simulink model "guidance_fuzzy_alt"  (R2017b)
settings: Solver=FixedStepDiscrete  StartTime=0.0  StopTime=inf  FixedStep=0.01  RelTol=1e-3
model workspace (MAT data in the model file):
  SL_ROS_VariableLengthArrays_MaxSizes : struct (value not decoded)
undefined symbols (not defined in the file): Data, Data_SL_Info
libraries: dspstat3 x14, robotlib x10, simulink_extras x7, simulink x4, dspswit3 x1
(part 2 of 2)

== system guidance_fuzzy_alt/pixel_per_sec_to_m_per_sec ==
  height : Inport
  vx(pix/sec) : Inport  Port=2
  vy(pix/sec) : Inport  Port=3
  Product : Product
  Product1 : Product
  camera_trigonometric_factor(m/pix) : Constant  Value=342.85
  of_vx_Divide : Product  Inputs=*/
  of_vy_Divide : Product  Inputs=*/
  vx_Moving Average : dspstat3/Moving Average  Method=Sliding window  SpecifyWindowLength=on  WindowLength=35  ForgettingFactor=0.9  SimulateUsing=Code generation
  vy_Moving Average : dspstat3/Moving Average  Method=Sliding window  SpecifyWindowLength=on  WindowLength=35  ForgettingFactor=0.9  SimulateUsing=Code generation
  vx(m/s) : Outport
  vy(m/s) : Outport  Port=2
  wires:
  height/1 -> Product1/1, Product/1
  of_vx_Divide/1 -> vx_Moving Average/1
  Product/1 -> of_vy_Divide/1
  Product1/1 -> of_vx_Divide/1
  vy_Moving Average/1 -> vy(m/s)/1
  vx_Moving Average/1 -> vx(m/s)/1
  of_vy_Divide/1 -> vy_Moving Average/1
  vy(pix/sec)/1 -> Product1/2
  camera_trigonometric_factor(m/pix)/1 -> of_vy_Divide/2, of_vx_Divide/2
  vx(pix/sec)/1 -> Product/2

== system guidance_fuzzy_alt/throttle_handler_climb_mode ==
  desired_throttle : Inport
  height : Inport  Port=2
  landing : Inport  Port=3
  If Action Subsystem4 : Subsystem  TreatAsAtomicUnit=on
  If Action Subsystem5 : Subsystem  TreatAsAtomicUnit=on
  If2 : If  IfExpression=u1 == 1  ElseIfExpressions=u1 == 0  ShowElse=off
  Merge2 : Merge
  Z_command : Scope
  throttle : Outport
  wires:
  height/1 -> If Action Subsystem4/1(In2)
  If Action Subsystem5/1(Out1) -> Merge2/2
  If Action Subsystem4/1(Out1) -> Merge2/1
  landing/1 -> If2/1
  Merge2/1 -> Z_command/1, throttle/1
  If2/1 -> If Action Subsystem4/Action
  If2/2 -> If Action Subsystem5/Action
  desired_throttle/1 -> If Action Subsystem5/1(In1)

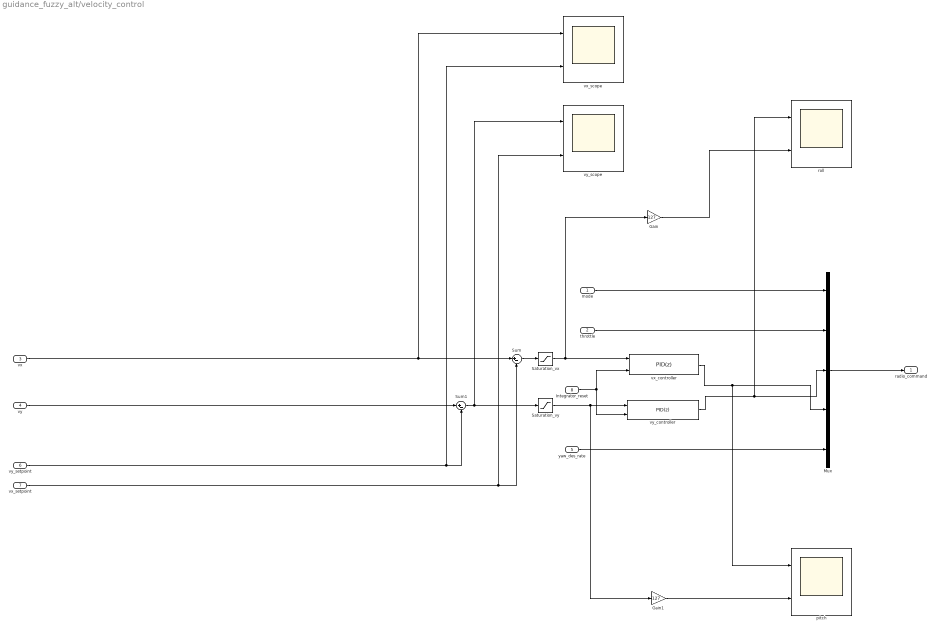
== system guidance_fuzzy_alt/velocity_control ==
  mode : Inport
  throttle : Inport  Port=2
  vx : Inport  Port=3
  vy : Inport  Port=4
  yaw_des_rate : Inport  Port=5
  vy_setpoint : Inport  Port=6
  vx_setpoint : Inport  Port=7
  Integrator_reset : Inport  Port=8
  Gain : Gain  Gain=127
  Gain1 : Gain  Gain=127
  Mux : Mux  Inputs=5
  Saturation_vx : Saturate  UpperLimit=1  LowerLimit=-1
  Saturation_vy : Saturate  UpperLimit=1  LowerLimit=-1
  Sum : Sum  Inputs=|+-
  Sum1 : Sum  Inputs=|+-
  pitch : Scope  NumInputPorts=2
  roll : Scope  NumInputPorts=2
  vx_controller : simulink/Continuous/PID Controller  Controller=PID  TimeDomain=Discrete-time  SampleTime=-1  IntegratorMethod=Forward Euler  FilterMethod=Forward Euler  Form=Parallel  UseFilter=on  ControllerParametersSource=internal  P=40  I=30  D=1  N=100  InitialConditionSource=internal  InitialConditionForIntegrator=0  InitialConditionForFilter=0  ExternalReset=either  LimitOutput=on  UpperSaturationLimit=127  LowerSaturationLimit=-127  LinearizeAsGain=off  AntiWindupMode=none  Kb=1  TrackingMode=off  Kt=1  PParamMin=[]  PParamMax=[]  IParamMin=[]  IParamMax=[]  DParamMin=[]  DParamMax=[]  NParamMin=[]  NParamMax=[]  KbParamMin=[]  KbParamMax=[]  KtParamMin=[]  KtParamMax=[]  POutMin=[]  POutMax=[]  IOutMin=[]  IOutMax=[]  DOutMin=[]  DOutMax=[]  NOutMin=[]  NOutMax=[]  KbOutMin=[]  KbOutMax=[]  KtOutMin=[]  KtOutMax=[]  IntegratorOutMin=[]  IntegratorOutMax=[]  FilterOutMin=[]  FilterOutMax=[]  SumOutMin=[]  SumOutMax=[]  SumI1OutMin=[]  SumI1OutMax=[]  SumI2OutMin=[]  SumI2OutMax=[]  SumI3OutMin=[]  SumI3OutMax=[]  SumDOutMin=[]  SumDOutMax=[]  SaturationOutMin=[]  SaturationOutMax=[]  IntegratorContinuousStateAttributes=''  IntegratorStateMustResolveToSignalObject=off  IntegratorRTWStateStorageClass=Auto  FilterContinuousStateAttributes=''  FilterStateMustResolveToSignalObject=off  FilterRTWStateStorageClass=Auto  DifferentiatorICPrevScaledInput=0  DifferentiatorOutMin=[]  DifferentiatorOutMax=[]  InitialConditionSetting=State (most efficient)  FilterDiffOutCoefMin=[]  FilterDiffOutCoefMax=[]  SumDenOutMin=[]  SumDenOutMax=[]  SumNumOutMin=[]  SumNumOutMax=[]  ReciprocalOutMin=[]  ReciprocalOutMax=[]  DivideOutMin=[]  DivideOutMax=[]  TunerSelectOption=Transfer Function Based (PID Tuner App)
  vx_scope : Scope  NumInputPorts=2
  vy_controller : simulink/Continuous/PID Controller  Controller=PID  TimeDomain=Discrete-time  SampleTime=-1  IntegratorMethod=Forward Euler  FilterMethod=Forward Euler  Form=Parallel  UseFilter=on  ControllerParametersSource=internal  P=40  I=30  D=1  N=100  InitialConditionSource=internal  InitialConditionForIntegrator=0  InitialConditionForFilter=0  ExternalReset=either  LimitOutput=on  UpperSaturationLimit=127  LowerSaturationLimit=-127  LinearizeAsGain=off  AntiWindupMode=none  Kb=1  TrackingMode=off  Kt=1  PParamMin=[]  PParamMax=[]  IParamMin=[]  IParamMax=[]  DParamMin=[]  DParamMax=[]  NParamMin=[]  NParamMax=[]  KbParamMin=[]  KbParamMax=[]  KtParamMin=[]  KtParamMax=[]  POutMin=[]  POutMax=[]  IOutMin=[]  IOutMax=[]  DOutMin=[]  DOutMax=[]  NOutMin=[]  NOutMax=[]  KbOutMin=[]  KbOutMax=[]  KtOutMin=[]  KtOutMax=[]  IntegratorOutMin=[]  IntegratorOutMax=[]  FilterOutMin=[]  FilterOutMax=[]  SumOutMin=[]  SumOutMax=[]  SumI1OutMin=[]  SumI1OutMax=[]  SumI2OutMin=[]  SumI2OutMax=[]  SumI3OutMin=[]  SumI3OutMax=[]  SumDOutMin=[]  SumDOutMax=[]  SaturationOutMin=[]  SaturationOutMax=[]  IntegratorContinuousStateAttributes=''  IntegratorStateMustResolveToSignalObject=off  IntegratorRTWStateStorageClass=Auto  FilterContinuousStateAttributes=''  FilterStateMustResolveToSignalObject=off  FilterRTWStateStorageClass=Auto  DifferentiatorICPrevScaledInput=0  DifferentiatorOutMin=[]  DifferentiatorOutMax=[]  InitialConditionSetting=State (most efficient)  FilterDiffOutCoefMin=[]  FilterDiffOutCoefMax=[]  SumDenOutMin=[]  SumDenOutMax=[]  SumNumOutMin=[]  SumNumOutMax=[]  ReciprocalOutMin=[]  ReciprocalOutMax=[]  DivideOutMin=[]  DivideOutMax=[]  TunerSelectOption=Transfer Function Based (PID Tuner App)
  vy_scope : Scope  NumInputPorts=2
  radio_command : Outport
  wires:
  vy/1 -> Sum1/1
  vy_setpoint/1 -> vx_scope/2, Sum1/2
  Sum1/1 -> Saturation_vy/1, vy_scope/1
  vy_controller/1 -> roll/1, Mux/3
  Mux/1 -> radio_command/1
  vx/1 -> vx_scope/1, Sum/1
  Sum/1 -> Saturation_vx/1
  vx_setpoint/1 -> vy_scope/2, Sum/2
  mode/1 -> Mux/1
  yaw_des_rate/1 -> Mux/5
  throttle/1 -> Mux/2
  vx_controller/1 -> pitch/1, Mux/4
  Integrator_reset/1 -> vy_controller/2, vx_controller/2
  Saturation_vx/1 -> Gain/1, vx_controller/1
  Saturation_vy/1 -> Gain1/1, vy_controller/1
  Gain/1 -> roll/2
  Gain1/1 -> pitch/2

== system guidance_fuzzy_alt/DataChangeTimer/If Action Subsystem ==
  In1 : Inport
  Action Port : ActionPort  ActionType=then
  Out1 : Outport
  wires:
  In1/1 -> Out1/1

== system guidance_fuzzy_alt/DataChangeTimer/If Action Subsystem1 ==
  In1 : Inport
  Action Port : ActionPort  ActionType=else
  Out1 : Outport
  wires:
  In1/1 -> Out1/1

== system guidance_fuzzy_alt/Subsystem/If Action Subsystem16 ==
  In1 : Inport
  Action Port : ActionPort  ActionType=else
  Out1 : Outport
  wires:
  In1/1 -> Out1/1

== system guidance_fuzzy_alt/Subsystem/If Action Subsystem9 ==
  In1 : Inport
  Action Port : ActionPort  ActionType=then
  Out1 : Outport
  wires:
  In1/1 -> Out1/1

== system guidance_fuzzy_alt/Subsystem/Switch Case Action Subsystem ==
  In1 : Inport
  Action Port : ActionPort  ActionType=case
  Out1 : Outport
  wires:
  In1/1 -> Out1/1

== system guidance_fuzzy_alt/Subsystem/Switch Case Action Subsystem1 ==
  In1 : Inport
  Action Port : ActionPort  ActionType=case
  Out1 : Outport
  wires:
  In1/1 -> Out1/1

== system guidance_fuzzy_alt/Subsystem/Switch Case Action Subsystem2 ==
  In1 : Inport
  Action Port : ActionPort  ActionType=case
  Out1 : Outport
  wires:
  In1/1 -> Out1/1

== system guidance_fuzzy_alt/Subsystem/Switch Case Action Subsystem3 ==
  In1 : Inport
  Action Port : ActionPort  ActionType=case
  Out1 : Outport
  wires:
  In1/1 -> Out1/1

== system guidance_fuzzy_alt/Subsystem2/If Action Subsystem ==
  In1 : Inport
  Action Port : ActionPort  ActionType=then
  Out1 : Outport
  wires:
  In1/1 -> Out1/1

== system guidance_fuzzy_alt/Subsystem2/If Action Subsystem1 ==
  In1 : Inport
  Action Port : ActionPort  ActionType=elseif
  Out1 : Outport
  wires:
  In1/1 -> Out1/1

== system guidance_fuzzy_alt/Subsystem2/If Action Subsystem2 ==
  In1 : Inport
  Action Port : ActionPort  ActionType=else
  Out1 : Outport
  wires:
  In1/1 -> Out1/1

== system guidance_fuzzy_alt/Subsystem5/If Action Subsystem2 ==
  In1 : Inport
  Action Port : ActionPort  ActionType=then
  Out1 : Outport
  wires:
  In1/1 -> Out1/1

== system guidance_fuzzy_alt/Subsystem5/If Action Subsystem3 ==
  In1 : Inport
  Action Port : ActionPort  ActionType=else
  Out1 : Outport
  wires:
  In1/1 -> Out1/1

== system guidance_fuzzy_alt/Subsystem6/If Action Subsystem1 ==
  In1 : Inport
  Action Port : ActionPort  ActionType=then
  Out1 : Outport
  wires:
  In1/1 -> Out1/1

== system guidance_fuzzy_alt/Subsystem6/If Action Subsystem10 ==
  In1 : Inport
  Action Port : ActionPort  ActionType=then
  Selector : Selector  InputPortWidth=128  IndexOptions=Index vector (dialog)  Indices=[1:8]  OutputSizes=1
  Out1 : Outport
  wires:
  In1/1 -> Selector/1
  Selector/1 -> Out1/1

== system guidance_fuzzy_alt/Subsystem6/If Action Subsystem11 ==
  In1 : Inport
  Action Port : ActionPort  ActionType=then
  Selector : Selector  InputPortWidth=128  IndexOptions=Index vector (dialog)  Indices=[1:16]  OutputSizes=1
  Out1 : Outport
  wires:
  In1/1 -> Selector/1
  Selector/1 -> Out1/1

== system guidance_fuzzy_alt/Subsystem6/If Action Subsystem12 ==
  In1 : Inport
  Action Port : ActionPort  ActionType=then
  Selector : Selector  InputPortWidth=128  IndexOptions=Index vector (dialog)  Indices=[1:24]  OutputSizes=1
  Out1 : Outport
  wires:
  In1/1 -> Selector/1
  Selector/1 -> Out1/1

== system guidance_fuzzy_alt/Subsystem6/If Action Subsystem13 ==
  In1 : Inport
  Action Port : ActionPort  ActionType=then
  Out1 : Outport
  wires:
  In1/1 -> Out1/1

== system guidance_fuzzy_alt/Subsystem6/If Action Subsystem14 ==
  In1 : Inport
  Action Port : ActionPort  ActionType=then
  Out1 : Outport
  wires:
  In1/1 -> Out1/1

== system guidance_fuzzy_alt/Subsystem6/If Action Subsystem15 ==
  In1 : Inport
  Action Port : ActionPort  ActionType=then
  Out1 : Outport
  wires:
  In1/1 -> Out1/1

== system guidance_fuzzy_alt/Subsystem6/If Action Subsystem4 ==
  In1 : Inport
  Action Port : ActionPort  ActionType=then
  Out1 : Outport
  wires:
  In1/1 -> Out1/1

== system guidance_fuzzy_alt/Subsystem6/If Action Subsystem5 ==
  In1 : Inport
  Action Port : ActionPort  ActionType=then
  Out1 : Outport
  wires:
  In1/1 -> Out1/1

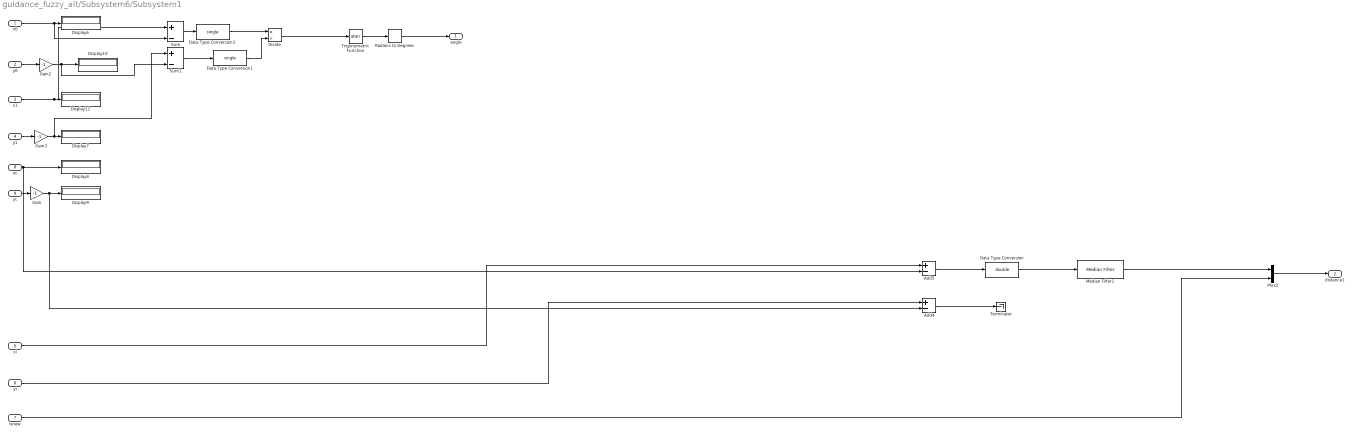
== system guidance_fuzzy_alt/Subsystem6/Subsystem1 ==
  x0 : Inport
  y0 : Inport  Port=2
  x1 : Inport  Port=3
  y1 : Inport  Port=4
  xi : Inport  Port=5
  yi : Inport  Port=6
  isnew : Inport  Port=7
  xc : Inport  Port=8
  yc : Inport  Port=9
  Add4 : Sum  Inputs=+-
  Add5 : Sum  Inputs=+-
  Data Type Conversion : DataTypeConversion  OutDataTypeStr=double
  Data Type Conversion1 : DataTypeConversion  OutDataTypeStr=single
  Data Type Conversion3 : DataTypeConversion  OutDataTypeStr=single
  Display{6..11} (6 alike) : Display
  Divide : Product  Inputs=*/
  Gain : Gain  Gain=-1
  Gain2 : Gain  Gain=-1
  Gain3 : Gain  Gain=-1
  Median Filter1 : dspstat3/Median Filter  WindowLength=20  SimulateUsing=Interpreted execution
      settings: SourceProductName=DSP System Toolbox  SourceProductBaseCode=DS
  Mux2 : Mux  Inputs=2
  Radians to Degrees : simulink_extras/Transformations/Radians to Degrees
  Sum : Sum  Inputs=|+-
  Sum1 : Sum  Inputs=|+-
  Terminator : Terminator
  Trigonometric Function : Trigonometry  Operator=atan
  angle : Outport
  distance1 : Outport  Port=2
  wires:
  x0/1 -> Sum/2, Display6/1
  Trigonometric Function/1 -> Radians to Degrees/1
  y0/1 -> Gain2/1
  Sum/1 -> Data Type Conversion3/1
  Gain3/1 -> Sum1/1, Display7/1
  Data Type Conversion3/1 -> Divide/1
  x1/1 -> Sum/1, Display11/1
  Add4/1 -> Terminator/1
  Gain/1 -> Display9/1, Add4/2
  yc/1 -> Gain/1
  Gain2/1 -> Sum1/2, Display10/1
  Add5/1 -> Data Type Conversion/1
  isnew/1 -> Mux2/2
  y1/1 -> Gain3/1
  xi/1 -> Add5/1
  Sum1/1 -> Data Type Conversion1/1
  Mux2/1 -> distance1/1
  Radians to Degrees/1 -> angle/1
  xc/1 -> Add5/2, Display8/1
  Divide/1 -> Trigonometric Function/1
  Data Type Conversion1/1 -> Divide/2
  Median Filter1/1 -> Mux2/1
  yi/1 -> Add4/1
  Data Type Conversion/1 -> Median Filter1/1

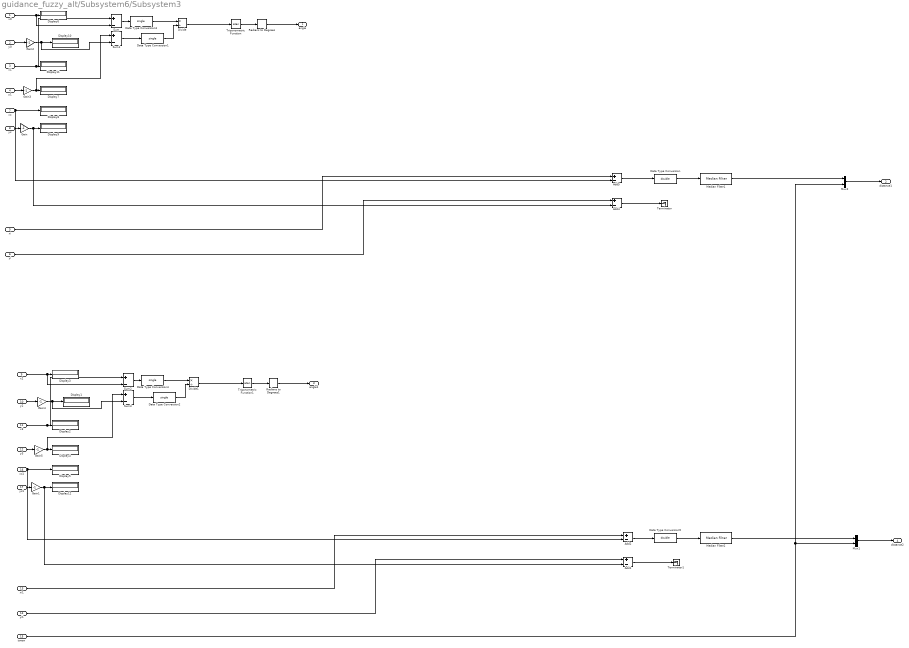
== system guidance_fuzzy_alt/Subsystem6/Subsystem3 ==
  x0 : Inport
  y0 : Inport  Port=2
  x1 : Inport  Port=3
  y1 : Inport  Port=4
  xi : Inport  Port=5
  yi : Inport  Port=6
  xc : Inport  Port=7
  yc : Inport  Port=8
  x2 : Inport  Port=9
  y2 : Inport  Port=10
  x3 : Inport  Port=11
  y3 : Inport  Port=12
  xi1 : Inport  Port=13
  yi1 : Inport  Port=14
  isnew : Inport  Port=15
  xc1 : Inport  Port=16
  yc1 : Inport  Port=17
  Add{1..2,4..5} (4 alike) : Sum  Inputs=+-
  Data Type Conversion : DataTypeConversion  OutDataTypeStr=double
  Data Type Conversion{1..4} (4 alike) : DataTypeConversion  OutDataTypeStr=single
  Data Type Conversion5 : DataTypeConversion  OutDataTypeStr=double
  Display{1..12} (12 alike) : Display
  Divide : Product  Inputs=*/
  Divide1 : Product  Inputs=*/
  Gain{,1..5} (6 alike) : Gain  Gain=-1
  Median Filter1 : dspstat3/Median Filter  WindowLength=20  SimulateUsing=Interpreted execution
      settings: SourceProductName=DSP System Toolbox  SourceProductBaseCode=DS
  Median Filter2 : dspstat3/Median Filter  WindowLength=20  SimulateUsing=Interpreted execution
      settings: SourceProductName=DSP System Toolbox  SourceProductBaseCode=DS
  Mux1 : Mux  Inputs=2
  Mux2 : Mux  Inputs=2
  Radians to Degrees : simulink_extras/Transformations/Radians to Degrees
  Radians to Degrees1 : simulink_extras/Transformations/Radians to Degrees
  Sum{,1..3} (4 alike) : Sum  Inputs=|+-
  Terminator : Terminator
  Terminator1 : Terminator
  Trigonometric Function : Trigonometry  Operator=atan
  Trigonometric Function1 : Trigonometry  Operator=atan
  angle : Outport
  distance1 : Outport  Port=2
  angle1 : Outport  Port=3
  distance2 : Outport  Port=4
  wires:
  Gain/1 -> Display9/1, Add4/2
  Divide/1 -> Trigonometric Function/1
  Data Type Conversion3/1 -> Divide/1
  Sum1/1 -> Data Type Conversion1/1
  Add4/1 -> Terminator/1
  x1/1 -> Sum/1, Display11/1
  Data Type Conversion1/1 -> Divide/2
  yc/1 -> Gain/1
  Radians to Degrees/1 -> angle/1
  y1/1 -> Gain3/1
  Gain2/1 -> Sum1/2, Display10/1
  Sum/1 -> Data Type Conversion3/1
  yi/1 -> Add4/1
  Add5/1 -> Data Type Conversion/1
  y0/1 -> Gain2/1
  xi/1 -> Add5/1
  Mux2/1 -> distance1/1
  Trigonometric Function/1 -> Radians to Degrees/1
  Gain3/1 -> Sum1/1, Display7/1
  Median Filter1/1 -> Mux2/1
  x0/1 -> Sum/2, Display6/1
  xc/1 -> Add5/2, Display8/1
  Gain1/1 -> Display12/1, Add1/2
  Divide1/1 -> Trigonometric Function1/1
  Data Type Conversion4/1 -> Divide1/1
  Sum3/1 -> Data Type Conversion2/1
  Add1/1 -> Terminator1/1
  x3/1 -> Sum2/1, Display2/1
  Data Type Conversion2/1 -> Divide1/2
  yc1/1 -> Gain1/1
  Radians to Degrees1/1 -> angle1/1
  y3/1 -> Gain5/1
  Gain4/1 -> Sum3/2, Display1/1
  isnew/1 -> Mux2/2, Mux1/2
  Sum2/1 -> Data Type Conversion4/1
  yi1/1 -> Add1/1
  Add2/1 -> Data Type Conversion5/1
  y2/1 -> Gain4/1
  xi1/1 -> Add2/1
  Mux1/1 -> distance2/1
  Trigonometric Function1/1 -> Radians to Degrees1/1
  Gain5/1 -> Sum3/1, Display4/1
  Median Filter2/1 -> Mux1/1
  x2/1 -> Sum2/2, Display3/1
  xc1/1 -> Add2/2, Display5/1
  Data Type Conversion/1 -> Median Filter1/1
  Data Type Conversion5/1 -> Median Filter2/1

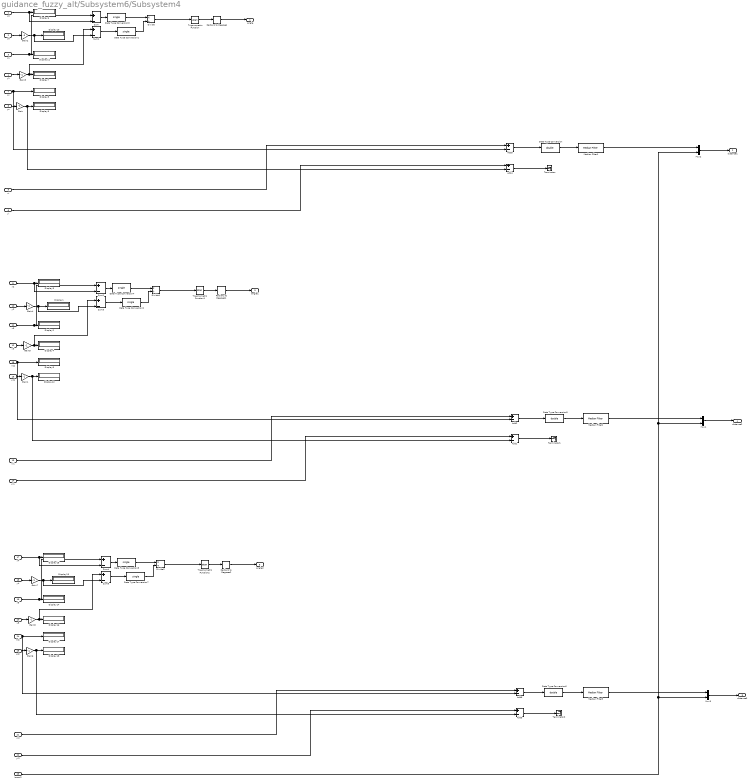
== system guidance_fuzzy_alt/Subsystem6/Subsystem4 ==
  x0 : Inport
  y0 : Inport  Port=2
  x1 : Inport  Port=3
  y1 : Inport  Port=4
  xi : Inport  Port=5
  yi : Inport  Port=6
  xc : Inport  Port=7
  yc : Inport  Port=8
  x2 : Inport  Port=9
  y2 : Inport  Port=10
  x3 : Inport  Port=11
  y3 : Inport  Port=12
  xi1 : Inport  Port=13
  yi1 : Inport  Port=14
  xc1 : Inport  Port=15
  yc1 : Inport  Port=16
  x4 : Inport  Port=17
  y4 : Inport  Port=18
  x5 : Inport  Port=19
  y5 : Inport  Port=20
  xi2 : Inport  Port=21
  yi2 : Inport  Port=22
  isnew2 : Inport  Port=23
  xc2 : Inport  Port=24
  yc2 : Inport  Port=25
  Add{1..6} (6 alike) : Sum  Inputs=+-
  Data Type Conversion : DataTypeConversion  OutDataTypeStr=double
  Data Type Conversion{1..4,7..8} (6 alike) : DataTypeConversion  OutDataTypeStr=single
  Data Type Conversion5 : DataTypeConversion  OutDataTypeStr=double
  Data Type Conversion6 : DataTypeConversion  OutDataTypeStr=double
  Display{1..18} (18 alike) : Display
  Divide : Product  Inputs=*/
  Divide1 : Product  Inputs=*/
  Divide2 : Product  Inputs=*/
  Gain{,1..8} (9 alike) : Gain  Gain=-1
  Median Filter1 : dspstat3/Median Filter  WindowLength=20  SimulateUsing=Interpreted execution
      settings: SourceProductName=DSP System Toolbox  SourceProductBaseCode=DS
  Median Filter2 : dspstat3/Median Filter  WindowLength=20  SimulateUsing=Interpreted execution
      settings: SourceProductName=DSP System Toolbox  SourceProductBaseCode=DS
  Median Filter3 : dspstat3/Median Filter  WindowLength=20  SimulateUsing=Interpreted execution
      settings: SourceProductName=DSP System Toolbox  SourceProductBaseCode=DS
  Mux1 : Mux  Inputs=2
  Mux2 : Mux  Inputs=2
  Mux3 : Mux  Inputs=2
  Radians to Degrees : simulink_extras/Transformations/Radians to Degrees
  Radians to Degrees1 : simulink_extras/Transformations/Radians to Degrees
  Radians to Degrees2 : simulink_extras/Transformations/Radians to Degrees
  Sum{,1..5} (6 alike) : Sum  Inputs=|+-
  Terminator : Terminator
  Terminator1 : Terminator
  Terminator2 : Terminator
  Trigonometric Function : Trigonometry  Operator=atan
  Trigonometric Function1 : Trigonometry  Operator=atan
  Trigonometric Function2 : Trigonometry  Operator=atan
  angle : Outport
  distance1 : Outport  Port=2
  angle1 : Outport  Port=3
  distance2 : Outport  Port=4
  angle2 : Outport  Port=5
  distance3 : Outport  Port=6
  wires:
  Gain/1 -> Display9/1, Add4/2
  Divide/1 -> Trigonometric Function/1
  Data Type Conversion3/1 -> Divide/1
  Sum1/1 -> Data Type Conversion1/1
  Add4/1 -> Terminator/1
  x1/1 -> Sum/1, Display11/1
  Data Type Conversion1/1 -> Divide/2
  yc/1 -> Gain/1
  Radians to Degrees/1 -> angle/1
  y1/1 -> Gain3/1
  Gain2/1 -> Sum1/2, Display10/1
  Sum/1 -> Data Type Conversion3/1
  yi/1 -> Add4/1
  Add5/1 -> Data Type Conversion/1
  y0/1 -> Gain2/1
  xi/1 -> Add5/1
  Mux2/1 -> distance1/1
  Trigonometric Function/1 -> Radians to Degrees/1
  Gain3/1 -> Sum1/1, Display7/1
  Median Filter1/1 -> Mux2/1
  x0/1 -> Sum/2, Display6/1
  xc/1 -> Add5/2, Display8/1
  Gain1/1 -> Display12/1, Add1/2
  Divide1/1 -> Trigonometric Function1/1
  Data Type Conversion4/1 -> Divide1/1
  Sum3/1 -> Data Type Conversion2/1
  Add1/1 -> Terminator1/1
  x3/1 -> Sum2/1, Display2/1
  Data Type Conversion2/1 -> Divide1/2
  yc1/1 -> Gain1/1
  Radians to Degrees1/1 -> angle1/1
  y3/1 -> Gain5/1
  Gain4/1 -> Sum3/2, Display1/1
  Sum2/1 -> Data Type Conversion4/1
  yi1/1 -> Add1/1
  Add2/1 -> Data Type Conversion5/1
  y2/1 -> Gain4/1
  xi1/1 -> Add2/1
  Mux1/1 -> distance2/1
  Trigonometric Function1/1 -> Radians to Degrees1/1
  Gain5/1 -> Sum3/1, Display4/1
  Median Filter2/1 -> Mux1/1
  x2/1 -> Sum2/2, Display3/1
  xc1/1 -> Add2/2, Display5/1
  Gain6/1 -> Display18/1, Add3/2
  Divide2/1 -> Trigonometric Function2/1
  Data Type Conversion8/1 -> Divide2/1
  Sum5/1 -> Data Type Conversion7/1
  Add3/1 -> Terminator2/1
  x5/1 -> Sum4/1, Display14/1
  Data Type Conversion7/1 -> Divide2/2
  yc2/1 -> Gain6/1
  Radians to Degrees2/1 -> angle2/1
  y5/1 -> Gain8/1
  Gain7/1 -> Sum5/2, Display13/1
  isnew2/1 -> Mux3/2, Mux1/2, Mux2/2
  Sum4/1 -> Data Type Conversion8/1
  yi2/1 -> Add3/1
  Add6/1 -> Data Type Conversion6/1
  y4/1 -> Gain7/1
  xi2/1 -> Add6/1
  Mux3/1 -> distance3/1
  Trigonometric Function2/1 -> Radians to Degrees2/1
  Gain8/1 -> Sum5/1, Display16/1
  Median Filter3/1 -> Mux3/1
  x4/1 -> Sum4/2, Display15/1
  xc2/1 -> Add6/2, Display17/1
  Data Type Conversion/1 -> Median Filter1/1
  Data Type Conversion5/1 -> Median Filter2/1
  Data Type Conversion6/1 -> Median Filter3/1

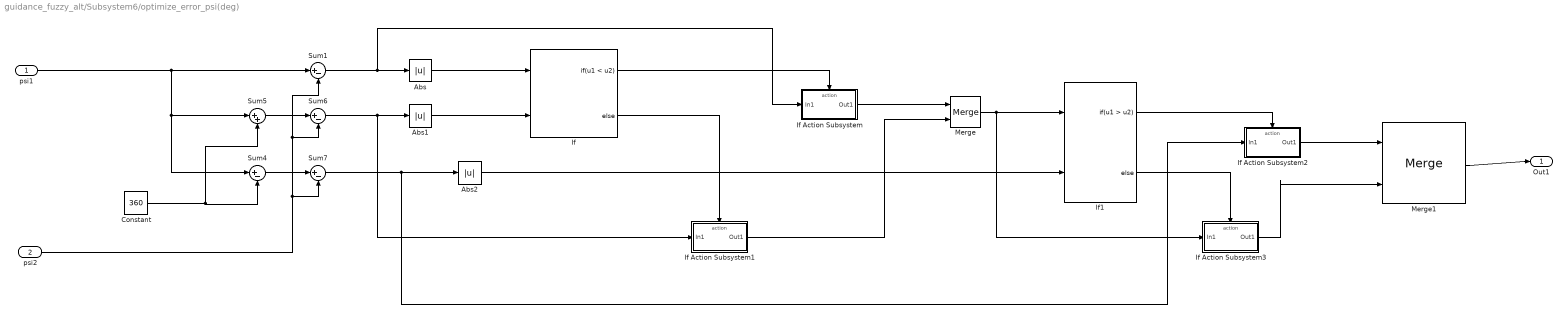
== system guidance_fuzzy_alt/Subsystem6/optimize_error_psi(deg) ==
  psi1 : Inport
  psi2 : Inport  Port=2
  Abs : Abs
  Abs1 : Abs
  Abs2 : Abs
  Constant : Constant  Value=360
  If : If  NumInputs=2  IfExpression=u1 < u2
  If Action Subsystem : Subsystem  TreatAsAtomicUnit=on
  If Action Subsystem1 : Subsystem  TreatAsAtomicUnit=on
  If Action Subsystem2 : Subsystem  TreatAsAtomicUnit=on
  If Action Subsystem3 : Subsystem  TreatAsAtomicUnit=on
  If1 : If  NumInputs=2  IfExpression=u1 > u2
  Merge : Merge
  Merge1 : Merge
  Sum{1,4,6..7} (4 alike) : Sum  Inputs=|+-
  Sum5 : Sum  Inputs=|++
  Out1 : Outport
  wires:
  Sum5/1 -> Sum6/1
  If Action Subsystem1/1(Out1) -> Merge/2
  Sum6/1 -> Abs1/1, If Action Subsystem1/1(In1)
  Abs/1 -> If/1
  If Action Subsystem/1(Out1) -> Merge/1
  If Action Subsystem2/1(Out1) -> Merge1/1
  Sum7/1 -> Abs2/1, If Action Subsystem2/1(In1)
  If/2 -> If Action Subsystem1/Action
  If/1 -> If Action Subsystem/Action
  Sum1/1 -> If Action Subsystem/1(In1), Abs/1
  Abs2/1 -> If1/2
  Merge/1 -> If1/1, If Action Subsystem3/1(In1)
  Merge1/1 -> Out1/1
  Abs1/1 -> If/2
  Sum4/1 -> Sum7/1
  Constant/1 -> Sum4/2, Sum5/2
  If1/2 -> If Action Subsystem3/Action
  If Action Subsystem3/1(Out1) -> Merge1/2
  If1/1 -> If Action Subsystem2/Action
  psi2/1 -> Sum1/2, Sum6/2, Sum7/2
  psi1/1 -> Sum4/1, Sum5/1, Sum1/1

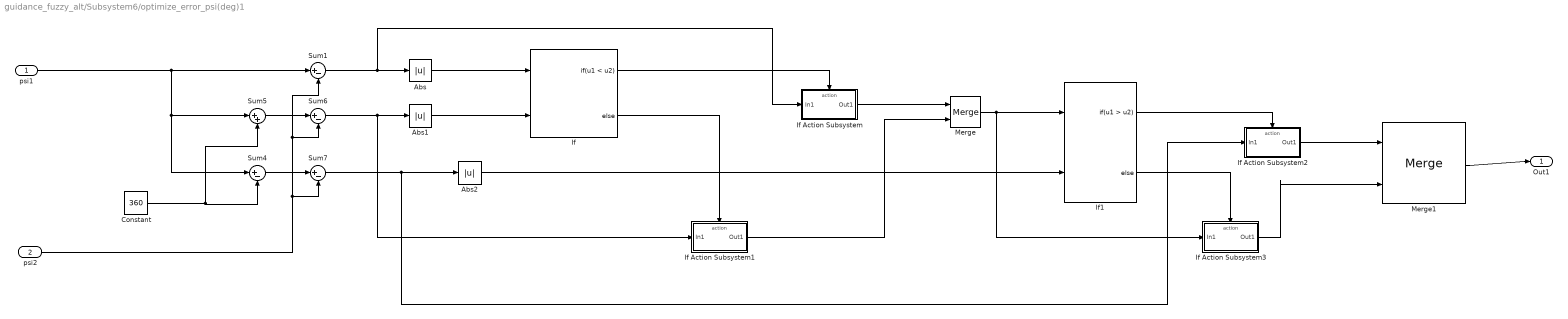
== system guidance_fuzzy_alt/Subsystem6/optimize_error_psi(deg)1 ==
  psi1 : Inport
  psi2 : Inport  Port=2
  Abs : Abs
  Abs1 : Abs
  Abs2 : Abs
  Constant : Constant  Value=360
  If : If  NumInputs=2  IfExpression=u1 < u2
  If Action Subsystem : Subsystem  TreatAsAtomicUnit=on
  If Action Subsystem1 : Subsystem  TreatAsAtomicUnit=on
  If Action Subsystem2 : Subsystem  TreatAsAtomicUnit=on
  If Action Subsystem3 : Subsystem  TreatAsAtomicUnit=on
  If1 : If  NumInputs=2  IfExpression=u1 > u2
  Merge : Merge
  Merge1 : Merge
  Sum{1,4,6..7} (4 alike) : Sum  Inputs=|+-
  Sum5 : Sum  Inputs=|++
  Out1 : Outport
  wires:
  psi1/1 -> Sum1/1, Sum5/1, Sum4/1
  psi2/1 -> Sum7/2, Sum6/2, Sum1/2
  If1/1 -> If Action Subsystem2/Action
  If Action Subsystem3/1(Out1) -> Merge1/2
  If1/2 -> If Action Subsystem3/Action
  Constant/1 -> Sum5/2, Sum4/2
  Sum4/1 -> Sum7/1
  Abs1/1 -> If/2
  Merge1/1 -> Out1/1
  Merge/1 -> If Action Subsystem3/1(In1), If1/1
  Abs2/1 -> If1/2
  Sum1/1 -> Abs/1, If Action Subsystem/1(In1)
  If/1 -> If Action Subsystem/Action
  If/2 -> If Action Subsystem1/Action
  Sum7/1 -> If Action Subsystem2/1(In1), Abs2/1
  If Action Subsystem2/1(Out1) -> Merge1/1
  If Action Subsystem/1(Out1) -> Merge/1
  Abs/1 -> If/1
  Sum6/1 -> If Action Subsystem1/1(In1), Abs1/1
  If Action Subsystem1/1(Out1) -> Merge/2
  Sum5/1 -> Sum6/1

== system guidance_fuzzy_alt/Subsystem6/optimize_error_psi(deg)2 ==
  psi1 : Inport
  psi2 : Inport  Port=2
  Abs : Abs
  Abs1 : Abs
  Abs2 : Abs
  Constant : Constant  Value=360
  If : If  NumInputs=2  IfExpression=u1 < u2
  If Action Subsystem : Subsystem  TreatAsAtomicUnit=on
  If Action Subsystem1 : Subsystem  TreatAsAtomicUnit=on
  If Action Subsystem2 : Subsystem  TreatAsAtomicUnit=on
  If Action Subsystem3 : Subsystem  TreatAsAtomicUnit=on
  If1 : If  NumInputs=2  IfExpression=u1 > u2
  Merge : Merge
  Merge1 : Merge
  Sum{1,4,6..7} (4 alike) : Sum  Inputs=|+-
  Sum5 : Sum  Inputs=|++
  Out1 : Outport
  wires:
  Sum5/1 -> Sum6/1
  If Action Subsystem1/1(Out1) -> Merge/2
  Sum6/1 -> Abs1/1, If Action Subsystem1/1(In1)
  Abs/1 -> If/1
  If Action Subsystem/1(Out1) -> Merge/1
  If Action Subsystem2/1(Out1) -> Merge1/1
  Sum7/1 -> Abs2/1, If Action Subsystem2/1(In1)
  If/2 -> If Action Subsystem1/Action
  If/1 -> If Action Subsystem/Action
  Sum1/1 -> If Action Subsystem/1(In1), Abs/1
  Abs2/1 -> If1/2
  Merge/1 -> If1/1, If Action Subsystem3/1(In1)
  Merge1/1 -> Out1/1
  Abs1/1 -> If/2
  Sum4/1 -> Sum7/1
  Constant/1 -> Sum4/2, Sum5/2
  If1/2 -> If Action Subsystem3/Action
  If Action Subsystem3/1(Out1) -> Merge1/2
  If1/1 -> If Action Subsystem2/Action
  psi2/1 -> Sum1/2, Sum6/2, Sum7/2
  psi1/1 -> Sum4/1, Sum5/1, Sum1/1

== system guidance_fuzzy_alt/Subsystem6/optimize_error_psi(deg)4 ==
  psi1 : Inport
  psi2 : Inport  Port=2
  Abs : Abs
  Abs1 : Abs
  Abs2 : Abs
  Constant : Constant  Value=360
  If : If  NumInputs=2  IfExpression=u1 < u2
  If Action Subsystem : Subsystem  TreatAsAtomicUnit=on
  If Action Subsystem1 : Subsystem  TreatAsAtomicUnit=on
  If Action Subsystem2 : Subsystem  TreatAsAtomicUnit=on
  If Action Subsystem3 : Subsystem  TreatAsAtomicUnit=on
  If1 : If  NumInputs=2  IfExpression=u1 > u2
  Merge : Merge
  Merge1 : Merge
  Sum{1,4,6..7} (4 alike) : Sum  Inputs=|+-
  Sum5 : Sum  Inputs=|++
  Out1 : Outport
  wires:
  psi1/1 -> Sum1/1, Sum5/1, Sum4/1
  psi2/1 -> Sum7/2, Sum6/2, Sum1/2
  If1/1 -> If Action Subsystem2/Action
  If Action Subsystem3/1(Out1) -> Merge1/2
  If1/2 -> If Action Subsystem3/Action
  Constant/1 -> Sum5/2, Sum4/2
  Sum4/1 -> Sum7/1
  Abs1/1 -> If/2
  Merge1/1 -> Out1/1
  Merge/1 -> If Action Subsystem3/1(In1), If1/1
  Abs2/1 -> If1/2
  Sum1/1 -> Abs/1, If Action Subsystem/1(In1)
  If/1 -> If Action Subsystem/Action
  If/2 -> If Action Subsystem1/Action
  Sum7/1 -> If Action Subsystem2/1(In1), Abs2/1
  If Action Subsystem2/1(Out1) -> Merge1/1
  If Action Subsystem/1(Out1) -> Merge/1
  Abs/1 -> If/1
  Sum6/1 -> If Action Subsystem1/1(In1), Abs1/1
  If Action Subsystem1/1(Out1) -> Merge/2
  Sum5/1 -> Sum6/1

== system guidance_fuzzy_alt/Subsystem6/optimize_error_psi(deg)5 ==
  psi1 : Inport
  psi2 : Inport  Port=2
  Abs : Abs
  Abs1 : Abs
  Abs2 : Abs
  Constant : Constant  Value=360
  If : If  NumInputs=2  IfExpression=u1 < u2
  If Action Subsystem : Subsystem  TreatAsAtomicUnit=on
  If Action Subsystem1 : Subsystem  TreatAsAtomicUnit=on
  If Action Subsystem2 : Subsystem  TreatAsAtomicUnit=on
  If Action Subsystem3 : Subsystem  TreatAsAtomicUnit=on
  If1 : If  NumInputs=2  IfExpression=u1 > u2
  Merge : Merge
  Merge1 : Merge
  Sum{1,4,6..7} (4 alike) : Sum  Inputs=|+-
  Sum5 : Sum  Inputs=|++
  Out1 : Outport
  wires:
  psi1/1 -> Sum1/1, Sum5/1, Sum4/1
  psi2/1 -> Sum7/2, Sum6/2, Sum1/2
  If1/1 -> If Action Subsystem2/Action
  If Action Subsystem3/1(Out1) -> Merge1/2
  If1/2 -> If Action Subsystem3/Action
  Constant/1 -> Sum5/2, Sum4/2
  Sum4/1 -> Sum7/1
  Abs1/1 -> If/2
  Merge1/1 -> Out1/1
  Merge/1 -> If Action Subsystem3/1(In1), If1/1
  Abs2/1 -> If1/2
  Sum1/1 -> Abs/1, If Action Subsystem/1(In1)
  If/1 -> If Action Subsystem/Action
  If/2 -> If Action Subsystem1/Action
  Sum7/1 -> If Action Subsystem2/1(In1), Abs2/1
  If Action Subsystem2/1(Out1) -> Merge1/1
  If Action Subsystem/1(Out1) -> Merge/1
  Abs/1 -> If/1
  Sum6/1 -> If Action Subsystem1/1(In1), Abs1/1
  If Action Subsystem1/1(Out1) -> Merge/2
  Sum5/1 -> Sum6/1

== system guidance_fuzzy_alt/Subsystem6/optimize_error_psi(deg)6 ==
  psi1 : Inport
  psi2 : Inport  Port=2
  Abs : Abs
  Abs1 : Abs
  Abs2 : Abs
  Constant : Constant  Value=360
  If : If  NumInputs=2  IfExpression=u1 < u2
  If Action Subsystem : Subsystem  TreatAsAtomicUnit=on
  If Action Subsystem1 : Subsystem  TreatAsAtomicUnit=on
  If Action Subsystem2 : Subsystem  TreatAsAtomicUnit=on
  If Action Subsystem3 : Subsystem  TreatAsAtomicUnit=on
  If1 : If  NumInputs=2  IfExpression=u1 > u2
  Merge : Merge
  Merge1 : Merge
  Sum{1,4,6..7} (4 alike) : Sum  Inputs=|+-
  Sum5 : Sum  Inputs=|++
  Out1 : Outport
  wires:
  psi1/1 -> Sum1/1, Sum5/1, Sum4/1
  psi2/1 -> Sum7/2, Sum6/2, Sum1/2
  If1/1 -> If Action Subsystem2/Action
  If Action Subsystem3/1(Out1) -> Merge1/2
  If1/2 -> If Action Subsystem3/Action
  Constant/1 -> Sum5/2, Sum4/2
  Sum4/1 -> Sum7/1
  Abs1/1 -> If/2
  Merge1/1 -> Out1/1
  Merge/1 -> If Action Subsystem3/1(In1), If1/1
  Abs2/1 -> If1/2
  Sum1/1 -> Abs/1, If Action Subsystem/1(In1)
  If/1 -> If Action Subsystem/Action
  If/2 -> If Action Subsystem1/Action
  Sum7/1 -> If Action Subsystem2/1(In1), Abs2/1
  If Action Subsystem2/1(Out1) -> Merge1/1
  If Action Subsystem/1(Out1) -> Merge/1
  Abs/1 -> If/1
  Sum6/1 -> If Action Subsystem1/1(In1), Abs1/1
  If Action Subsystem1/1(Out1) -> Merge/2
  Sum5/1 -> Sum6/1

== system guidance_fuzzy_alt/attitude_failsafe/If Action Subsystem ==
  Action Port : ActionPort  ActionType=then

== system guidance_fuzzy_alt/attitude_failsafe/If Action Subsystem1 ==
  Action Port : ActionPort  ActionType=else
  Constant : Constant
  Data Store Write : DataStoreWrite  DataStoreName=kill
  wires:
  Constant/1 -> Data Store Write/1

== system guidance_fuzzy_alt/attitude_failsafe/If Action Subsystem2 ==
  In1 : Inport
  Action Port : ActionPort  ActionType=then
  Out1 : Outport
  wires:
  In1/1 -> Out1/1

== system guidance_fuzzy_alt/attitude_failsafe/If Action Subsystem3 ==
  In1 : Inport
  Action Port : ActionPort  ActionType=else
  Out1 : Outport
  wires:
  In1/1 -> Out1/1

== system guidance_fuzzy_alt/attitude_failsafe/If Action Subsystem4 ==
  Action Port : ActionPort  ActionType=then
  Constant : Constant  Value=0
  Data Store Write : DataStoreWrite  DataStoreName=kill
  wires:
  Constant/1 -> Data Store Write/1

== system guidance_fuzzy_alt/check_arm_status/If Action Subsystem1 ==
  In1 : Inport
  Action Port : ActionPort  ActionType=then
  Out1 : Outport
  wires:
  In1/1 -> Out1/1

== system guidance_fuzzy_alt/check_arm_status/If Action Subsystem2 ==
  In1 : Inport
  Action Port : ActionPort  ActionType=elseif
  Out1 : Outport
  wires:
  In1/1 -> Out1/1

== system guidance_fuzzy_alt/check_arm_status/If Action Subsystem3 ==
  In1 : Inport
  Action Port : ActionPort  ActionType=else
  Out1 : Outport
  wires:
  In1/1 -> Out1/1

== system guidance_fuzzy_alt/command_input/DataChangeTimer ==
  trig : Inport
  Abs : Abs
  Data Type Conversion : DataTypeConversion  OutDataTypeStr=uint8
  Digital Clock : DigitalClock  SampleTime=0.01
  If : If
  If Action Subsystem : Subsystem  TreatAsAtomicUnit=on
  If Action Subsystem1 : Subsystem  TreatAsAtomicUnit=on
  Subtract : Sum  Inputs=+-
  diff_time : Outport
  wires:
  If Action Subsystem1/1(Out1) -> Subtract/2
  Subtract/1 -> Abs/1
  trig/1 -> Data Type Conversion/1
  Abs/1 -> diff_time/1
  If Action Subsystem/1(Out1) -> Subtract/1
  Digital Clock/1 -> If Action Subsystem1/1(In1), If Action Subsystem/1(In1)
  If/2 -> If Action Subsystem1/Action
  If/1 -> If Action Subsystem/Action
  Data Type Conversion/1 -> If/1

== system guidance_fuzzy_alt/command_input/If Action Subsystem2 ==
  In1 : Inport
  Action Port : ActionPort  ActionType=then
  Out1 : Outport
  wires:
  In1/1 -> Out1/1

== system guidance_fuzzy_alt/command_input/If Action Subsystem3 ==
  In1 : Inport
  Action Port : ActionPort  ActionType=else
  Out1 : Outport
  wires:
  In1/1 -> Out1/1

== system guidance_fuzzy_alt/optimize_error_psi(deg)1/If Action Subsystem ==
  In1 : Inport
  Action Port : ActionPort  ActionType=then
  Out1 : Outport
  wires:
  In1/1 -> Out1/1

== system guidance_fuzzy_alt/optimize_error_psi(deg)1/If Action Subsystem1 ==
  In1 : Inport
  Action Port : ActionPort  ActionType=else
  Out1 : Outport
  wires:
  In1/1 -> Out1/1

== system guidance_fuzzy_alt/optimize_error_psi(deg)1/If Action Subsystem2 ==
  In1 : Inport
  Action Port : ActionPort  ActionType=then
  Out1 : Outport
  wires:
  In1/1 -> Out1/1

== system guidance_fuzzy_alt/optimize_error_psi(deg)1/If Action Subsystem3 ==
  In1 : Inport
  Action Port : ActionPort  ActionType=else
  Out1 : Outport
  wires:
  In1/1 -> Out1/1

== system guidance_fuzzy_alt/optimize_error_psi(deg)3/If Action Subsystem ==
  In1 : Inport
  Action Port : ActionPort  ActionType=then
  Out1 : Outport
  wires:
  In1/1 -> Out1/1

== system guidance_fuzzy_alt/optimize_error_psi(deg)3/If Action Subsystem1 ==
  In1 : Inport
  Action Port : ActionPort  ActionType=else
  Out1 : Outport
  wires:
  In1/1 -> Out1/1

== system guidance_fuzzy_alt/optimize_error_psi(deg)3/If Action Subsystem2 ==
  In1 : Inport
  Action Port : ActionPort  ActionType=then
  Out1 : Outport
  wires:
  In1/1 -> Out1/1

== system guidance_fuzzy_alt/optimize_error_psi(deg)3/If Action Subsystem3 ==
  In1 : Inport
  Action Port : ActionPort  ActionType=else
  Out1 : Outport
  wires:
  In1/1 -> Out1/1

== system guidance_fuzzy_alt/throttle_handler_climb_mode/If Action Subsystem4 ==
  In2 : Inport
  Action Port : ActionPort  ActionType=then
  Constant1 : Constant  Value=0
  Constant4 : Constant  Value=47
  If : If  IfExpression=u1 < 0.1
  If Action Subsystem : Subsystem  TreatAsAtomicUnit=on
  If Action Subsystem1 : Subsystem  TreatAsAtomicUnit=on
  Merge : Merge
  Out1 : Outport
  wires:
  Merge/1 -> Out1/1
  If/1 -> If Action Subsystem/Action
  If/2 -> If Action Subsystem1/Action
  Constant1/1 -> If Action Subsystem/1(In1)
  In2/1 -> If/1
  Constant4/1 -> If Action Subsystem1/1(In1)
  If Action Subsystem/1(Out1) -> Merge/1
  If Action Subsystem1/1(Out1) -> Merge/2

== system guidance_fuzzy_alt/throttle_handler_climb_mode/If Action Subsystem5 ==
  In1 : Inport
  Action Port : ActionPort  ActionType=elseif
  Data Type Conversion : DataTypeConversion  OutDataTypeStr=double
  Out1 : Outport
  wires:
  In1/1 -> Data Type Conversion/1
  Data Type Conversion/1 -> Out1/1

== system guidance_fuzzy_alt/Subsystem6/optimize_error_psi(deg)/If Action Subsystem ==
  In1 : Inport
  Action Port : ActionPort  ActionType=then
  Out1 : Outport
  wires:
  In1/1 -> Out1/1

== system guidance_fuzzy_alt/Subsystem6/optimize_error_psi(deg)/If Action Subsystem1 ==
  In1 : Inport
  Action Port : ActionPort  ActionType=else
  Out1 : Outport
  wires:
  In1/1 -> Out1/1

== system guidance_fuzzy_alt/Subsystem6/optimize_error_psi(deg)/If Action Subsystem2 ==
  In1 : Inport
  Action Port : ActionPort  ActionType=then
  Out1 : Outport
  wires:
  In1/1 -> Out1/1

== system guidance_fuzzy_alt/Subsystem6/optimize_error_psi(deg)/If Action Subsystem3 ==
  In1 : Inport
  Action Port : ActionPort  ActionType=else
  Out1 : Outport
  wires:
  In1/1 -> Out1/1

== system guidance_fuzzy_alt/Subsystem6/optimize_error_psi(deg)1/If Action Subsystem ==
  In1 : Inport
  Action Port : ActionPort  ActionType=then
  Out1 : Outport
  wires:
  In1/1 -> Out1/1

== system guidance_fuzzy_alt/Subsystem6/optimize_error_psi(deg)1/If Action Subsystem1 ==
  In1 : Inport
  Action Port : ActionPort  ActionType=else
  Out1 : Outport
  wires:
  In1/1 -> Out1/1

== system guidance_fuzzy_alt/Subsystem6/optimize_error_psi(deg)1/If Action Subsystem2 ==
  In1 : Inport
  Action Port : ActionPort  ActionType=then
  Out1 : Outport
  wires:
  In1/1 -> Out1/1

== system guidance_fuzzy_alt/Subsystem6/optimize_error_psi(deg)1/If Action Subsystem3 ==
  In1 : Inport
  Action Port : ActionPort  ActionType=else
  Out1 : Outport
  wires:
  In1/1 -> Out1/1

== system guidance_fuzzy_alt/Subsystem6/optimize_error_psi(deg)2/If Action Subsystem ==
  In1 : Inport
  Action Port : ActionPort  ActionType=then
  Out1 : Outport
  wires:
  In1/1 -> Out1/1

== system guidance_fuzzy_alt/Subsystem6/optimize_error_psi(deg)2/If Action Subsystem1 ==
  In1 : Inport
  Action Port : ActionPort  ActionType=else
  Out1 : Outport
  wires:
  In1/1 -> Out1/1

== system guidance_fuzzy_alt/Subsystem6/optimize_error_psi(deg)2/If Action Subsystem2 ==
  In1 : Inport
  Action Port : ActionPort  ActionType=then
  Out1 : Outport
  wires:
  In1/1 -> Out1/1

== system guidance_fuzzy_alt/Subsystem6/optimize_error_psi(deg)2/If Action Subsystem3 ==
  In1 : Inport
  Action Port : ActionPort  ActionType=else
  Out1 : Outport
  wires:
  In1/1 -> Out1/1

== system guidance_fuzzy_alt/Subsystem6/optimize_error_psi(deg)4/If Action Subsystem ==
  In1 : Inport
  Action Port : ActionPort  ActionType=then
  Out1 : Outport
  wires:
  In1/1 -> Out1/1

== system guidance_fuzzy_alt/Subsystem6/optimize_error_psi(deg)4/If Action Subsystem1 ==
  In1 : Inport
  Action Port : ActionPort  ActionType=else
  Out1 : Outport
  wires:
  In1/1 -> Out1/1

== system guidance_fuzzy_alt/Subsystem6/optimize_error_psi(deg)4/If Action Subsystem2 ==
  In1 : Inport
  Action Port : ActionPort  ActionType=then
  Out1 : Outport
  wires:
  In1/1 -> Out1/1

== system guidance_fuzzy_alt/Subsystem6/optimize_error_psi(deg)4/If Action Subsystem3 ==
  In1 : Inport
  Action Port : ActionPort  ActionType=else
  Out1 : Outport
  wires:
  In1/1 -> Out1/1

== system guidance_fuzzy_alt/Subsystem6/optimize_error_psi(deg)5/If Action Subsystem ==
  In1 : Inport
  Action Port : ActionPort  ActionType=then
  Out1 : Outport
  wires:
  In1/1 -> Out1/1

== system guidance_fuzzy_alt/Subsystem6/optimize_error_psi(deg)5/If Action Subsystem1 ==
  In1 : Inport
  Action Port : ActionPort  ActionType=else
  Out1 : Outport
  wires:
  In1/1 -> Out1/1

== system guidance_fuzzy_alt/Subsystem6/optimize_error_psi(deg)5/If Action Subsystem2 ==
  In1 : Inport
  Action Port : ActionPort  ActionType=then
  Out1 : Outport
  wires:
  In1/1 -> Out1/1

== system guidance_fuzzy_alt/Subsystem6/optimize_error_psi(deg)5/If Action Subsystem3 ==
  In1 : Inport
  Action Port : ActionPort  ActionType=else
  Out1 : Outport
  wires:
  In1/1 -> Out1/1

== system guidance_fuzzy_alt/Subsystem6/optimize_error_psi(deg)6/If Action Subsystem ==
  In1 : Inport
  Action Port : ActionPort  ActionType=then
  Out1 : Outport
  wires:
  In1/1 -> Out1/1

== system guidance_fuzzy_alt/Subsystem6/optimize_error_psi(deg)6/If Action Subsystem1 ==
  In1 : Inport
  Action Port : ActionPort  ActionType=else
  Out1 : Outport
  wires:
  In1/1 -> Out1/1

== system guidance_fuzzy_alt/Subsystem6/optimize_error_psi(deg)6/If Action Subsystem2 ==
  In1 : Inport
  Action Port : ActionPort  ActionType=then
  Out1 : Outport
  wires:
  In1/1 -> Out1/1

== system guidance_fuzzy_alt/Subsystem6/optimize_error_psi(deg)6/If Action Subsystem3 ==
  In1 : Inport
  Action Port : ActionPort  ActionType=else
  Out1 : Outport
  wires:
  In1/1 -> Out1/1

== system guidance_fuzzy_alt/command_input/DataChangeTimer/If Action Subsystem ==
  In1 : Inport
  Action Port : ActionPort  ActionType=then
  Out1 : Outport
  wires:
  In1/1 -> Out1/1

== system guidance_fuzzy_alt/command_input/DataChangeTimer/If Action Subsystem1 ==
  In1 : Inport
  Action Port : ActionPort  ActionType=else
  Out1 : Outport
  wires:
  In1/1 -> Out1/1

== system guidance_fuzzy_alt/throttle_handler_climb_mode/If Action Subsystem4/If Action Subsystem ==
  In1 : Inport
  Action Port : ActionPort  ActionType=then
  Constant : Constant
  Data Store Write : DataStoreWrite  DataStoreName=kill
  Out1 : Outport
  wires:
  In1/1 -> Out1/1
  Constant/1 -> Data Store Write/1

== system guidance_fuzzy_alt/throttle_handler_climb_mode/If Action Subsystem4/If Action Subsystem1 ==
  In1 : Inport
  Action Port : ActionPort  ActionType=else
  Out1 : Outport
  wires:
  In1/1 -> Out1/1
